simulink library "allActuatorCtrl_cl"  (R2018b)
settings: Solver=VariableStepAuto  StartTime=0.0  StopTime=10.0  RelTol=1e-3
values from neighbouring files (symbols this model uses):
  ctrl = allActuatorCtrlClass    [allActuatorCtrl_ts.m]    (also in compareScalingResults.m)
libraries: filteredPIDController_ul x5
settings Model: Creator=mcobb  LastModifiedBy=mcobb

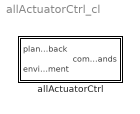
== system allActuatorCtrl_cl ==
  allActuatorCtrl : Subsystem

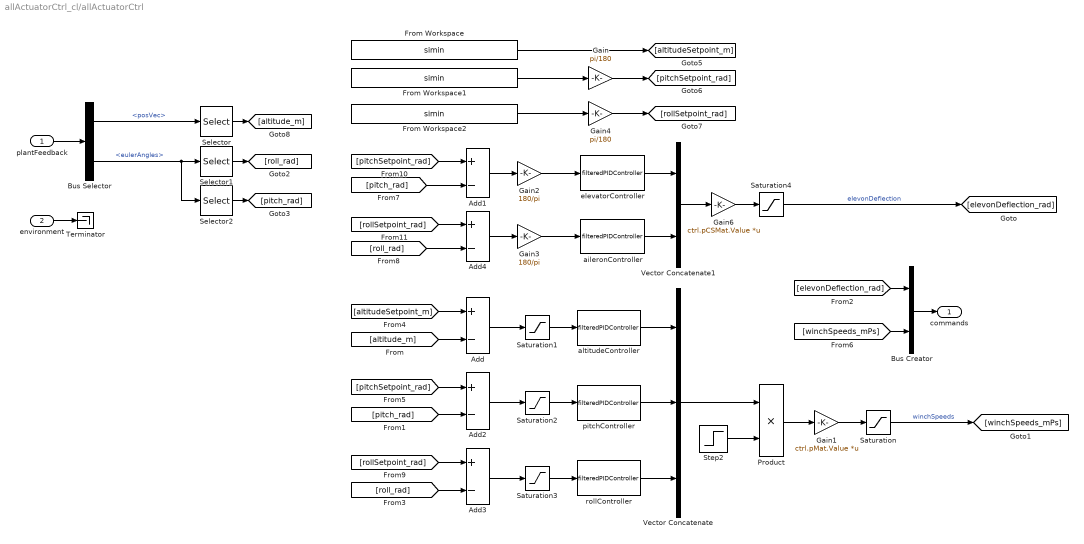
== system allActuatorCtrl_cl/allActuatorCtrl ==
  plantFeedback : Inport  OutDataTypeStr=Bus: plantBus
  environment : Inport  Port=2  OutDataTypeStr=Bus: envBus
  Add{,1..4} (5 alike) : Sum  Inputs=+-
  Bus Creator : BusCreator  Inputs=2
  Bus Selector : BusSelector  OutputSignals=posVec,eulerAngles
  From Workspace : FromWorkspace  VariableName=simin  SampleTime=0
  From Workspace1 : FromWorkspace  VariableName=simin  SampleTime=0
  From Workspace2 : FromWorkspace  VariableName=simin  SampleTime=0
  Gain : Gain  Gain=pi/180
  Gain1 : Gain  Gain=ctrl.pMat.Value  Multiplication=Matrix(K*u)
  Gain2 : Gain  Gain=180/pi
  Gain3 : Gain  Gain=180/pi
  Gain4 : Gain  Gain=pi/180
  Gain6 : Gain  Gain=ctrl.pCSMat.Value  Multiplication=Matrix(K*u)
  Product : Product
  Saturation : Saturate  UpperLimit=ctrl.winchSpeedCmdLim.Value  LowerLimit=-ctrl.winchSpeedCmdLim.Value
  Saturation1 : Saturate  UpperLimit=5  LowerLimit=-5
  Saturation2 : Saturate  UpperLimit=5  LowerLimit=-5
  Saturation3 : Saturate  UpperLimit=5  LowerLimit=-5
  Saturation4 : Saturate  UpperLimit=ctrl.elevonMaxDeflection.Value*pi/180  LowerLimit=-ctrl.elevonMaxDeflection.Value*pi/180
  Selector : Selector  InputPortWidth=3  IndexOptions=Index vector (dialog)  Indices=3  OutputSizes=1
  Selector1 : Selector  InputPortWidth=3  IndexOptions=Index vector (dialog)  Indices=1  OutputSizes=1
  Selector2 : Selector  InputPortWidth=3  IndexOptions=Index vector (dialog)  Indices=2  OutputSizes=1
  Step2 : Step  Time=0  SampleTime=0
  Terminator : Terminator
  Vector Concatenate : Concatenate  NumInputs=3
  Vector Concatenate1 : Concatenate
  aileronController : filteredPIDController_ul/filteredPIDController  kp=ctrl.aileronKp.Value  ki=ctrl.aileronKi.Value  kd=ctrl.aileronKd.Value  tau=ctrl.aileronFilterTimeConst.Value
  altitudeController : filteredPIDController_ul/filteredPIDController  kp=ctrl.altitudeKp.Value  ki=ctrl.altitudeKi.Value  kd=ctrl.altitudeKd.Value  tau=ctrl.altitudeFilterTimeConst.Value
  elevatorController : filteredPIDController_ul/filteredPIDController  kp=ctrl.elevatorKp.Value  ki=ctrl.elevatorKi.Value  kd=ctrl.elevatorKd.Value  tau=ctrl.elevatorFilterTimeConst.Value
  pitchController : filteredPIDController_ul/filteredPIDController  kp=ctrl.pitchKp.Value  ki=ctrl.pitchKi.Value  kd=ctrl.pitchKd.Value  tau=ctrl.pitchFilterTimeConst.Value
  rollController : filteredPIDController_ul/filteredPIDController  kp=ctrl.rollKp.Value  ki=ctrl.rollKi.Value  kd=ctrl.rollKd.Value  tau=ctrl.rollFilterTimeConst.Value
  commands : Outport  OutDataTypeStr=Bus: ctrlBus
  wires:
  Product/1 -> Gain1/1
  Step2/1 -> Product/2
  Vector Concatenate/1 -> Product/1
  Gain1/1 -> Saturation/1
  Saturation2/1 -> pitchController/1
  Saturation3/1 -> rollController/1
  Saturation1/1 -> altitudeController/1
  [pitchSetpoint_rad] -> Add2/1
  [pitch_rad] -> Add2/2
  [roll_rad] -> Add3/2
  [rollSetpoint_rad] -> Add3/1
  rollController/1 -> Vector Concatenate/3
  Add2/1 -> Saturation2/1
  [altitude_m] -> Add/2
  [altitudeSetpoint_m] -> Add/1
  Add/1 -> Saturation1/1
  pitchController/1 -> Vector Concatenate/2
  altitudeController/1 -> Vector Concatenate/1
  Add3/1 -> Saturation3/1
  Saturation4/1 -> [elevonDeflection_rad]  "elevonDeflection"
  Vector Concatenate1/1 -> Gain6/1
  aileronController/1 -> Vector Concatenate1/2
  elevatorController/1 -> Vector Concatenate1/1
  [roll_rad] -> Add4/2
  Add4/1 -> Gain3/1
  [pitch_rad] -> Add1/2
  Gain6/1 -> Saturation4/1
  Gain2/1 -> elevatorController/1
  Gain3/1 -> aileronController/1
  Add1/1 -> Gain2/1
  Bus Creator/1 -> commands/1
  Saturation/1 -> [winchSpeeds_mPs]  "winchSpeeds"
  [elevonDeflection_rad] -> Bus Creator/1
  [winchSpeeds_mPs] -> Bus Creator/2
  environment/1 -> Terminator/1
  plantFeedback/1 -> Bus Selector/1
  Gain/1 -> [pitchSetpoint_rad]
  Gain4/1 -> [rollSetpoint_rad]
  Selector/1 -> [altitude_m]
  [pitchSetpoint_rad] -> Add1/1
  [rollSetpoint_rad] -> Add4/1
  Bus Selector/1 -> Selector/1  "<posVec>"
  Bus Selector/2 -> Selector2/1, Selector1/1  "<eulerAngles>"
  Selector1/1 -> [roll_rad]
  Selector2/1 -> [pitch_rad]
  From Workspace/1 -> [altitudeSetpoint_m]
  From Workspace1/1 -> Gain/1
  From Workspace2/1 -> Gain4/1
